simulink library "sselecpowersrclib"  (R2015a)
settings: Solver=ode45  StartTime=0.0  StopTime=10.0  RelTol=1e-3
libraries: fl_lib x3
settings Model: Creator=e102261  LastModifiedBy=e102261
settings DataIOCC: SaveOutput=off  SignalLogging=off  DSMLogging=off  VisualizeSimOutput=off  SaveTime=off

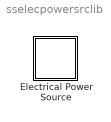
== system sselecpowersrclib ==
  Electrical Power Source : Subsystem  mask(Electrical Power Source){}
      mask help: This block allows the user to deliver a specified electrical power to an electrical circuit. It automatically adjusts the current so that the power product p(t) = i(t) x v(t) is correct. Note that you will encounter problems if v(t) falls to or passes through zero. This block has been written with energy storage elements such as batteries and supercapacitors in mind. Users are responsible for ensuring that this block is suitable for their applications.
      mask Display:
      | disp('P')
      | plot(0.5+0.3*sin(linspace(0,2*pi,36)), 0.5+0.3*cos(linspace(0,2*pi,36)))
      | plot([0.5 0.5], [0.8 1])
      | plot([0 1 1 0 0],[1 1 0 0 1]);
      | plot([0.25 0.25 0.5 0.5], [0 0.1 0.1 0.2]);
      | color('red');
      | port_label('RConn', 1, '+')
      | port_label('LConn', 1, 'P')
      | port_label('LConn', 2, '-')

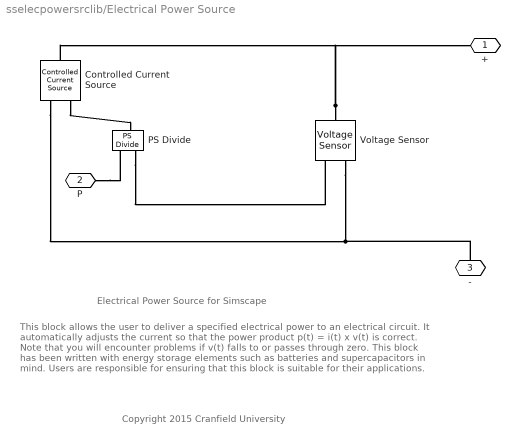
== system sselecpowersrclib/Electrical Power Source ==
  note: Electrical Power Source for Simscape
  note: Copyright 2015 Cranfield University
  note: This block allows the user to deliver a specified electrical power to an electrical
      | circuit. It automatically adjusts the current so that the power product
      | p(t) = i(t) x v(t) is correct.  Note that you will encounter problems if v(t) falls to or
      | passes through zero. This block has been written with energy storage elements
      | such as batteries and supercapacitors in mind. Users are responsible for
      | ensuring that this block is suitable for their applications.
  Controlled Current Source : fl_lib/Electrical/Electrical Sources/Controlled Current Source
  PS Divide : fl_lib/Physical Signals/Functions/PS Divide
  Voltage Sensor : fl_lib/Electrical/Electrical Sensors/Voltage Sensor
  + : PMIOPort  Port=1  Side=Right
  P : PMIOPort  Port=2  Side=Left
  - : PMIOPort  Port=3  Side=Left
  connections:
  PS Divide/LConn2 -- Voltage Sensor/RConn1
  P/RConn1 -- PS Divide/LConn1
  Controlled Current Source/RConn1 -- PS Divide/RConn1
  Voltage Sensor/LConn1 -- +/RConn1 -- Controlled Current Source/LConn1
  -/RConn1 -- Voltage Sensor/RConn2 -- Controlled Current Source/RConn2
